simulink model "trajectory"  (R2017b)
settings: Solver=ode4  StartTime=0.0  StopTime=T  FixedStep=dt  RelTol=1e-3
values from neighbouring files (symbols this model uses):
  acc_noise = ( 3 /3*0.01)^2*dt *1    (= 1e-06)    [gene_traj.m]
  gyro_noise = ( 0.1 /3/180*pi)^2*dt *1    (= 3.38463799763e-09)    [gene_traj.m]
undefined symbols (not defined in the file or in its folder): att0
libraries: aerolibconvert2 x2, aerolibutil x2, sharedtransform x2, shared6dof x1, aerolibnav x1, simulink x1
settings Model: Creator=longteng  LastModifiedBy=longteng
settings Model: ModifiedComment=|
  | longteng -- Fri Jan 19 20:51:12 2018 -- Version 1.2
  | Exchange position and velocity output.
settings Model: ModifiedHistory=|
  | longteng -- Fri Jan 19 20:51:12 2018 -- Version 1.2
  | Exchange position and velocity output.
  | 
  | longteng -- Fri Jan 19 20:31:53 2018 -- Version 1.1
  | Create model.
settings DataIOCC: SaveOutput=off  SignalLogging=off  DSMLogging=off  SaveTime=off

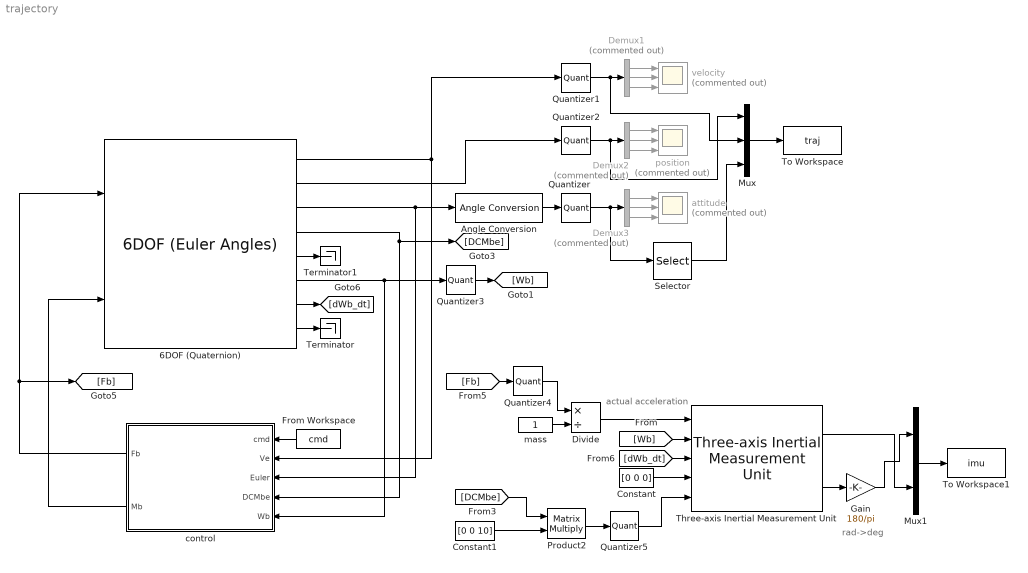
== system trajectory ==
  note: rad->deg
  note: actual acceleration
  6DOF (Quaternion) : shared6dof/6DOF (Euler Angles)  units=Metric (MKS)  mtype=Fixed  rep=Quaternion  xme_0=[0 0 0]  Vm_0=vb0  eul_0=[att0(3) att0(2) att0(1)]/180*pi  pm_0=[0 0 0]  mass_0=1.0  mass_e=0.5  mass_f=2.0  inertia=eye(3)  inertia_e=eye(3)  inertia_f=2*eye(3)  k_quat=1.0  vre_flag=on  abi_flag=off
      settings: SourceProductBaseCode=AE
  Angle Conversion : aerolibconvert2/Angle Conversion  IU=rad  OU=deg
  Constant : Constant  Value=[0 0 0]
  Constant1 : Constant  Value=[0 0 10]
  Demux1 : Demux  Commented=on  Outputs=3
  Demux2 : Demux  Commented=on  Outputs=3
  Demux3 : Demux  Commented=on  Outputs=3
  Divide : Product  Inputs=*/
  From Workspace : FromWorkspace  VariableName=cmd  SampleTime=0  OutputAfterFinalValue=Setting to zero
  Gain : Gain  Gain=180/pi
  Mux : Mux  Inputs=3
  Mux1 : Mux  Inputs=2
  Product2 : Product  Multiplication=Matrix(*)
  Quantizer : Quantizer  QuantizationInterval=1e-4
  Quantizer1 : Quantizer  QuantizationInterval=0.001
  Quantizer2 : Quantizer  QuantizationInterval=0.001
  Quantizer3 : Quantizer  QuantizationInterval=1e-12
  Quantizer4 : Quantizer  QuantizationInterval=1e-12
  Quantizer5 : Quantizer  QuantizationInterval=1e-12
  Selector : Selector  InputPortWidth=3  IndexOptions=Index vector (dialog)  Indices=[3 2 1]  OutputSizes=1
  Terminator : Terminator
  Terminator1 : Terminator
  Three-axis Inertial Measurement Unit : aerolibnav/Three-axis Inertial Measurement Unit  units=Metric (MKS)  imu=[0 0 0]  i_Ts=dt  dtype_a=off  w_a=190  z_a=0.707  a_sf_cc=[1 0 0; 0 1 0; 0 0 1]  a_bias=acc_bias  a_sat="[-inf  -inf  -inf  inf inf inf]"  dtype_g=off  w_g=190  z_g=0.707  g_sf_cc=[1 0 0; 0 1 0; 0 0 1]  g_bias=gyro_bias  g_sens=[0 0 0]  g_sat="[-inf  -inf  -inf  inf inf inf]"  i_rand=on  i_seeds=noise_seeds  i_pow=[acc_noise*ones(1,3),gyro_noise*ones(1,3)]
  To Workspace : ToWorkspace  VariableName=traj  SampleTime=-1
  To Workspace1 : ToWorkspace  VariableName=imu  SampleTime=-1
  attitude : Scope  Commented=on  NumInputPorts=3
  control : Subsystem
  mass : Constant
  position : Scope  Commented=on  NumInputPorts=3
  velocity : Scope  Commented=on  NumInputPorts=3
  wires:
  6DOF (Quaternion)/3 -> Angle Conversion/1, control/3(Euler)
  6DOF (Quaternion)/6 -> Quantizer3/1, control/5(Wb)
  control/1(Fb) -> [Fb], 6DOF (Quaternion)/1
  control/2(Mb) -> 6DOF (Quaternion)/2
  6DOF (Quaternion)/8 -> Terminator/1
  Angle Conversion/1 -> Quantizer/1
  Demux3/3 -> attitude/3
  Demux3/2 -> attitude/2
  Demux3/1 -> attitude/1
  Demux1/3 -> velocity/3
  Demux1/1 -> velocity/1
  Demux1/2 -> velocity/2
  6DOF (Quaternion)/1 -> control/2(Ve), Quantizer1/1
  6DOF (Quaternion)/5 -> Terminator1/1
  Demux2/1 -> position/1
  Demux2/2 -> position/2
  Demux2/3 -> position/3
  6DOF (Quaternion)/2 -> Quantizer2/1
  From Workspace/1 -> control/1(cmd)
  Mux/1 -> To Workspace/1
  Quantizer/1 -> Selector/1, Demux3/1
  Quantizer2/1 -> Mux/1, Demux2/1
  Quantizer1/1 -> Mux/2, Demux1/1
  6DOF (Quaternion)/7 -> [dWb_dt]
  Three-axis Inertial Measurement Unit/2 -> Gain/1
  mass/1 -> Divide/2
  Divide/1 -> Three-axis Inertial Measurement Unit/1
  [dWb_dt] -> Three-axis Inertial Measurement Unit/3
  Constant/1 -> Three-axis Inertial Measurement Unit/4
  [Wb] -> Three-axis Inertial Measurement Unit/2
  [Fb] -> Quantizer4/1
  Mux1/1 -> To Workspace1/1
  Constant1/1 -> Product2/2
  Product2/1 -> Quantizer5/1
  6DOF (Quaternion)/4 -> control/4(DCMbe), [DCMbe]
  Three-axis Inertial Measurement Unit/1 -> Mux1/2
  Gain/1 -> Mux1/1
  Quantizer3/1 -> [Wb]
  Quantizer4/1 -> Divide/1
  [DCMbe] -> Product2/1
  Quantizer5/1 -> Three-axis Inertial Measurement Unit/5
  Selector/1 -> Mux/3

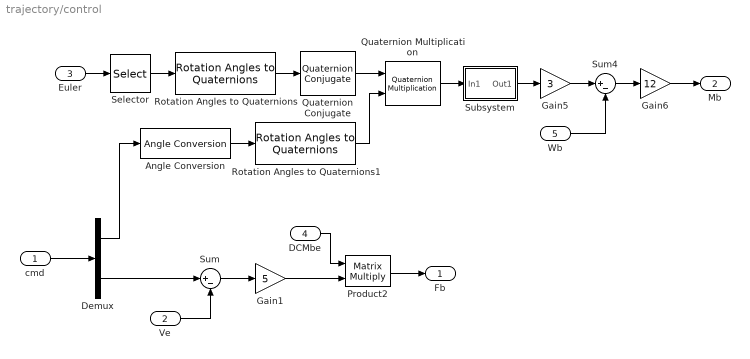
== system trajectory/control ==
  cmd : Inport
  Ve : Inport  Port=2
  Euler : Inport  Port=3
  DCMbe : Inport  Port=4
  Wb : Inport  Port=5
  Angle Conversion : aerolibconvert2/Angle Conversion  IU=deg  OU=rad
  Demux : Demux  Outputs=[3 3]
  Gain1 : Gain  Gain=5
  Gain5 : Gain  Gain=3
  Gain6 : Gain  Gain=12
  Product2 : Product  Multiplication=Matrix(*)
  Quaternion Conjugate : aerolibutil/Quaternion Conjugate
      settings: SourceProductName=Aerospace Blockset  SourceProductBaseCode=AE
  Quaternion Multiplication : aerolibutil/Quaternion Multiplication
  Rotation Angles to Quaternions : sharedtransform/Rotation Angles to Quaternions  rotationOrder=ZYX
      settings: SourceProductName=Aerospace Blockset  SourceProductBaseCode=AE
  Rotation Angles to Quaternions1 : sharedtransform/Rotation Angles to Quaternions  rotationOrder=ZYX
      settings: SourceProductName=Aerospace Blockset  SourceProductBaseCode=AE
  Selector : Selector  InputPortWidth=3  IndexOptions=Index vector (dialog)  Indices=[3 2 1]  OutputSizes=1
  Subsystem : Subsystem
  Sum : Sum  Inputs=|+-
  Sum4 : Sum  Inputs=|+-
  Fb : Outport
  Mb : Outport  Port=2
  wires:
  cmd/1 -> Demux/1
  Subsystem/1(Out1) -> Gain5/1
  Rotation Angles to Quaternions/1 -> Quaternion Conjugate/1
  Euler/1 -> Selector/1
  Quaternion Multiplication/1 -> Subsystem/1(In1)
  Rotation Angles to Quaternions1/1 -> Quaternion Multiplication/2
  Quaternion Conjugate/1 -> Quaternion Multiplication/1
  Angle Conversion/1 -> Rotation Angles to Quaternions1/1
  Selector/1 -> Rotation Angles to Quaternions/1
  Demux/1 -> Angle Conversion/1
  Sum4/1 -> Gain6/1
  Gain5/1 -> Sum4/1
  Wb/1 -> Sum4/2
  Gain6/1 -> Mb/1
  Demux/2 -> Sum/1
  Ve/1 -> Sum/2
  Sum/1 -> Gain1/1
  Gain1/1 -> Product2/2
  DCMbe/1 -> Product2/1
  Product2/1 -> Fb/1

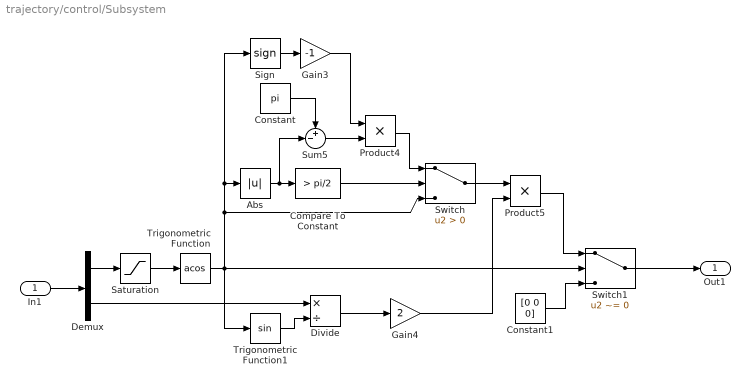
== system trajectory/control/Subsystem ==
  In1 : Inport
  Abs : Abs
  Compare To Constant : simulink/Logic and Bit Operations/Compare To Constant  relop=>  const=pi/2  OutDataTypeStr=boolean
  Constant : Constant  Value=pi
  Constant1 : Constant  Value=[0 0 0]
  Demux : Demux  Outputs=[1 3]
  Divide : Product  Inputs=*/
  Gain3 : Gain  Gain=-1
  Gain4 : Gain  Gain=2
  Product4 : Product
  Product5 : Product
  Saturation : Saturate  UpperLimit=1  LowerLimit=-1
  Sign : Signum
  Sum5 : Sum  Inputs=+-|
  Switch : Switch  Criteria=u2 > Threshold
  Switch1 : Switch  Criteria=u2 ~= 0
  Trigonometric Function : Trigonometry  Operator=acos
  Trigonometric Function1 : Trigonometry
  Out1 : Outport
  wires:
  Demux/1 -> Saturation/1
  In1/1 -> Demux/1
  Gain3/1 -> Product4/1
  Constant/1 -> Sum5/1
  Trigonometric Function/1 -> Trigonometric Function1/1, Switch1/2, Sign/1, Abs/1, Switch/3
  Abs/1 -> Sum5/2, Compare To Constant/1
  Constant1/1 -> Switch1/3
  Switch1/1 -> Out1/1
  Switch/1 -> Product5/1
  Gain4/1 -> Product5/2
  Trigonometric Function1/1 -> Divide/2
  Demux/2 -> Divide/1
  Divide/1 -> Gain4/1
  Product5/1 -> Switch1/1
  Sign/1 -> Gain3/1
  Compare To Constant/1 -> Switch/2
  Product4/1 -> Switch/1
  Sum5/1 -> Product4/2
  Saturation/1 -> Trigonometric Function/1
